simulink model "Lev_project_control_coop_obs"  (R2022b)
settings: Solver=VariableStepAuto  StartTime=0.0  StopTime=Tsim  FixedStep=0.001  RelTol=1e-3
values from neighbouring files (symbols this model uses):
  A = A-B*K0    [project.m]
  Ad = zeros(6,6)    [project.m]
  B = [0; -9.9453]    [project.m]
  C = [708.27 0]    [project.m]
  c = 1/(2*real(minimum_eig))    [project.m]
  D = 0    [project.m]
  G = diag([0 1 0 6 0 0])    [project.m]
  K = (R\B')*P    [project.m]
  x_0 = [0 0]'    [project.m]
  x_0_Leader = [0 2]'    [project.m]
undefined symbols (not defined in the file or in its folder): observer
libraries: matrix_library x6
settings Model: Creator=Matteo  LastModifiedBy=Soff

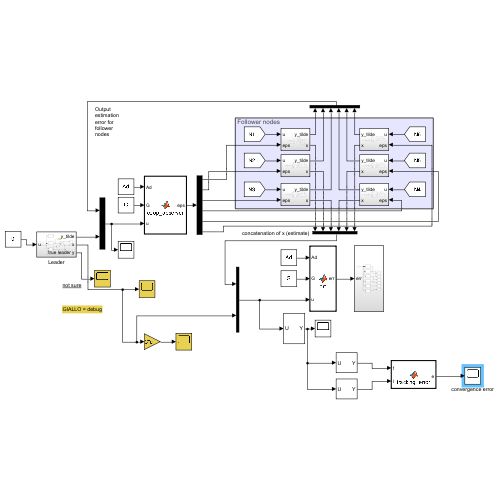
[thumbnail: Simulink's stored preview of the top-level diagram]
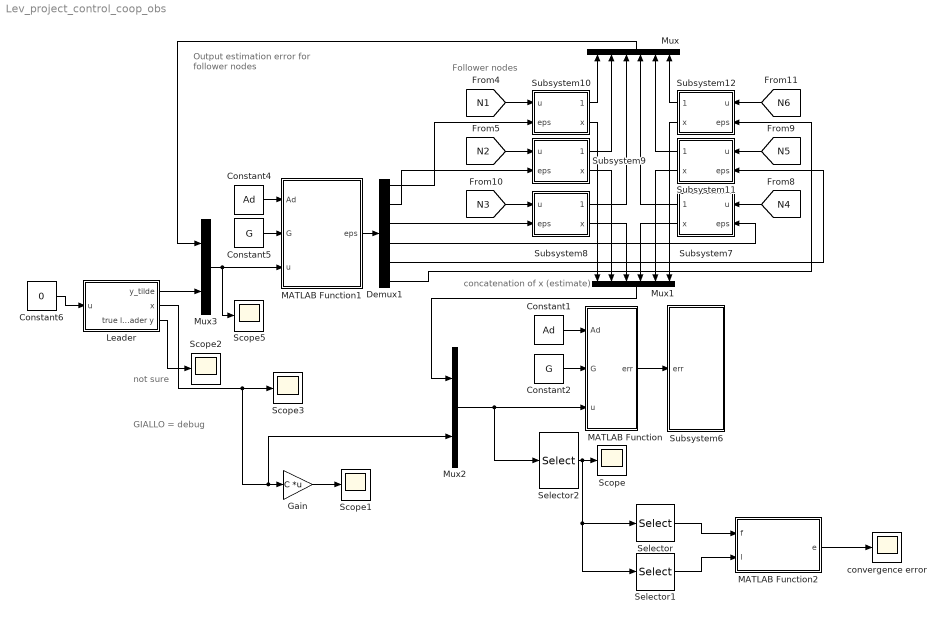
== system Lev_project_control_coop_obs ==
  note: GIALLO = debug
  note: concatenation of x (estimate)
  note: Follower nodes
  note: not sure
  note: Output estimation error for follower nodes
  Constant1 : Constant  Value=Ad
  Constant2 : Constant  Value=G
  Constant4 : Constant  Value=Ad
  Constant5 : Constant  Value=G
  Constant6 : Constant  Value=0
  Demux1 : Demux  Outputs=6
  Gain : Gain  Gain=C  Multiplication=Matrix(K*u)
  Leader : Subsystem
  MATLAB Function : MATLAB Function  TreatAsAtomicUnit=on
  MATLAB Function1 : MATLAB Function  TreatAsAtomicUnit=on
  MATLAB Function2 : MATLAB Function  TreatAsAtomicUnit=on
  Mux : Mux  Inputs=6
  Mux1 : Mux  Inputs=6
  Mux2 : Mux  Inputs=2
  Mux3 : Mux  Inputs=2
  Scope{,1..3,5} (5 alike) : Scope
  Selector : Selector  InputPortWidth=7  IndexOptions=Index vector (dialog)  Indices=[1 2 3 4 5 6]  OutputSizes=1
  Selector1 : Selector  InputPortWidth=7  IndexOptions=Index vector (dialog)  Indices=[7]  OutputSizes=1
  Selector2 : Selector  InputPortWidth=14  IndexOptions=Index vector (dialog)  Indices=[1 3 5 7 9 11 13]  OutputSizes=1
  Subsystem10 : Subsystem
  Subsystem11 : Subsystem
  Subsystem12 : Subsystem
  Subsystem6 : Subsystem
  Subsystem7 : Subsystem
  Subsystem8 : Subsystem
  Subsystem9 : Subsystem
  convergence error : Scope
  wires:
  Constant1/1 -> MATLAB Function/1(Ad)
  Constant2/1 -> MATLAB Function/2(G)
  Constant4/1 -> MATLAB Function1/1(Ad)
  Constant5/1 -> MATLAB Function1/2(G)
  MATLAB Function1/1(eps) -> Demux1/1
  Constant6/1 -> Leader/1(u)
  Mux3/1 -> Scope5/1, MATLAB Function1/3(u)
  Leader/2(x) -> Mux2/2, Gain/1, Scope3/1
  Mux2/1 -> Selector2/1, MATLAB Function/3(u)
  Gain/1 -> Scope1/1
  Leader/3(true leader y) -> Scope2/1
  MATLAB Function/1(err) -> Subsystem6/1(err)
  [N1] -> Subsystem10/1(u)
  [N4] -> Subsystem7/1(u)
  [N2] -> Subsystem9/1(u)
  [N3] -> Subsystem8/1(u)
  [N5] -> Subsystem11/1(u)
  [N6] -> Subsystem12/1(u)
  Subsystem10/1(y_tilde) -> Mux/1
  Subsystem9/1(y_tilde) -> Mux/2
  Subsystem8/1(y_tilde) -> Mux/3
  Subsystem12/1(y_tilde) -> Mux/6
  Subsystem11/1(y_tilde) -> Mux/5
  Subsystem7/1(y_tilde) -> Mux/4
  Demux1/1 -> Subsystem10/2(eps)
  Demux1/3 -> Subsystem8/2(eps)
  Mux/1 -> Mux3/1
  Subsystem10/2(x) -> Mux1/1
  Subsystem9/2(x) -> Mux1/2
  Subsystem8/2(x) -> Mux1/3
  Subsystem7/2(x) -> Mux1/4
  Subsystem11/2(x) -> Mux1/5
  Subsystem12/2(x) -> Mux1/6
  Mux1/1 -> Mux2/1
  Demux1/2 -> Subsystem9/2(eps)
  Demux1/4 -> Subsystem7/2(eps)
  Demux1/5 -> Subsystem11/2(eps)
  Demux1/6 -> Subsystem12/2(eps)
  Leader/1(y_tilde) -> Mux3/2
  Selector2/1 -> Selector/1, Selector1/1, Scope/1
  MATLAB Function2/1(e) -> convergence error/1
  Selector1/1 -> MATLAB Function2/2(l)
  Selector/1 -> MATLAB Function2/1(f)

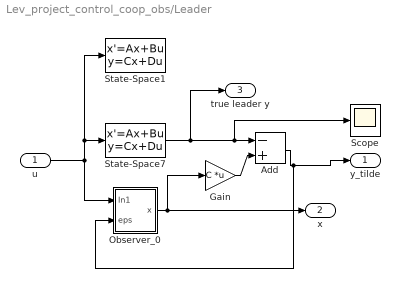
== system Lev_project_control_coop_obs/Leader ==
  u : Inport
  Add : Sum  Inputs=-+
  Gain : Gain  Gain=C  Multiplication=Matrix(K*u)
  Observer_0 : Subsystem
  Scope : Scope
  State-Space1 : StateSpace  A=A  B=B  C=eye(2)  D=zeros(2,1)  InitialCondition=x_0_Leader
  State-Space7 : StateSpace  A=A  B=B  C=C  D=D  InitialCondition=x_0_Leader
  y_tilde : Outport
  x : Outport  Port=2
  true leader y : Outport  Port=3
  wires:
  State-Space7/1 -> Scope/1, Add/1, true leader y/1
  u/1 -> State-Space1/1, State-Space7/1, Observer_0/1(In1)
  Add/1 -> Observer_0/2(eps), y_tilde/1
  Gain/1 -> Add/2
  Observer_0/1(x) -> x/1, Gain/1

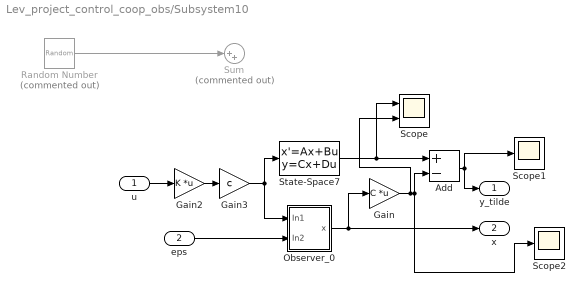
== system Lev_project_control_coop_obs/Subsystem10 ==
  u : Inport
  eps : Inport  Port=2
  Add : Sum  Inputs=+-
  Gain : Gain  Gain=C  Multiplication=Matrix(K*u)
  Gain2 : Gain  Gain=K  Multiplication=Matrix(K*u)
  Gain3 : Gain  Gain=c
  Observer_0 : Subsystem
  Random Number : RandomNumber  Commented=on  SampleTime=0.1
  Scope : Scope  NumInputPorts=2
  Scope1 : Scope
  Scope2 : Scope
  State-Space7 : StateSpace  A=A  B=B  C=C  D=D  InitialCondition=x_0
  Sum : Sum  Commented=on  Inputs=|++
  y_tilde : Outport
  x : Outport  Port=2
  wires:
  Gain/1 -> Scope/2, Add/2, Scope2/1
  Add/1 -> y_tilde/1, Scope1/1
  eps/1 -> Observer_0/2(In2)
  Observer_0/1(x) -> x/1, Gain/1
  u/1 -> Gain2/1
  Gain2/1 -> Gain3/1
  Gain3/1 -> Observer_0/1(In1), State-Space7/1
  Random Number/1 -> Sum/1
  State-Space7/1 -> Scope/1, Add/1

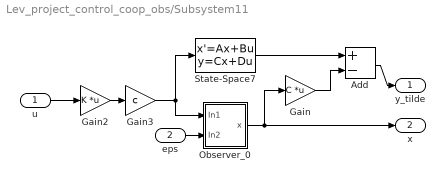
== system Lev_project_control_coop_obs/Subsystem11 ==
  u : Inport
  eps : Inport  Port=2
  Add : Sum  Inputs=+-
  Gain : Gain  Gain=C  Multiplication=Matrix(K*u)
  Gain2 : Gain  Gain=K  Multiplication=Matrix(K*u)
  Gain3 : Gain  Gain=c
  Observer_0 : Subsystem
  State-Space7 : StateSpace  A=A  B=B  C=C  D=D  InitialCondition=x_0
  y_tilde : Outport
  x : Outport  Port=2
  wires:
  u/1 -> Gain2/1
  Add/1 -> y_tilde/1
  Gain/1 -> Add/2
  State-Space7/1 -> Add/1
  Observer_0/1(x) -> x/1, Gain/1
  eps/1 -> Observer_0/2(In2)
  Gain2/1 -> Gain3/1
  Gain3/1 -> Observer_0/1(In1), State-Space7/1

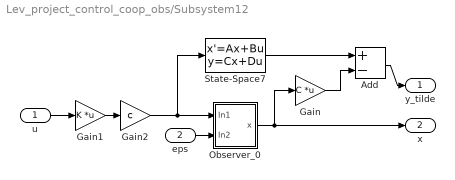
== system Lev_project_control_coop_obs/Subsystem12 ==
  u : Inport
  eps : Inport  Port=2
  Add : Sum  Inputs=+-
  Gain : Gain  Gain=C  Multiplication=Matrix(K*u)
  Gain1 : Gain  Gain=K  Multiplication=Matrix(K*u)
  Gain2 : Gain  Gain=c
  Observer_0 : Subsystem
  State-Space7 : StateSpace  A=A  B=B  C=C  D=D  InitialCondition=x_0
  y_tilde : Outport
  x : Outport  Port=2
  wires:
  Add/1 -> y_tilde/1
  Gain/1 -> Add/2
  State-Space7/1 -> Add/1
  Observer_0/1(x) -> x/1, Gain/1
  eps/1 -> Observer_0/2(In2)
  Gain1/1 -> Gain2/1
  Gain2/1 -> Observer_0/1(In1), State-Space7/1
  u/1 -> Gain1/1

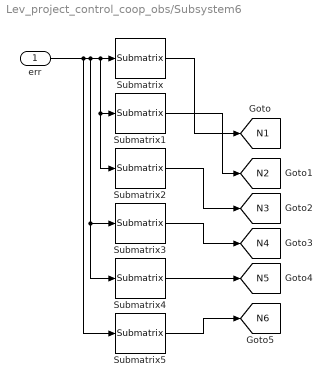
== system Lev_project_control_coop_obs/Subsystem6 ==
  err : Inport
  Submatrix : matrix_library/Submatrix  RowSpan=All rows  RowStartMode=First  RowStartIndex=1  RowEndMode=Last  RowEndIndex=1  ColSpan=One column  ColStartMode=Index  ColStartIndex=1  ColEndMode=Last  ColEndIndex=1
  Submatrix1 : matrix_library/Submatrix  RowSpan=All rows  RowStartMode=First  RowStartIndex=1  RowEndMode=Last  RowEndIndex=1  ColSpan=One column  ColStartMode=Index  ColStartIndex=2  ColEndMode=Last  ColEndIndex=1
  Submatrix2 : matrix_library/Submatrix  RowSpan=All rows  RowStartMode=First  RowStartIndex=1  RowEndMode=Last  RowEndIndex=1  ColSpan=One column  ColStartMode=Index  ColStartIndex=3  ColEndMode=Last  ColEndIndex=1
  Submatrix3 : matrix_library/Submatrix  RowSpan=All rows  RowStartMode=First  RowStartIndex=1  RowEndMode=Last  RowEndIndex=1  ColSpan=One column  ColStartMode=Index  ColStartIndex=4  ColEndMode=Last  ColEndIndex=1
  Submatrix4 : matrix_library/Submatrix  RowSpan=All rows  RowStartMode=First  RowStartIndex=1  RowEndMode=Last  RowEndIndex=1  ColSpan=One column  ColStartMode=Index  ColStartIndex=5  ColEndMode=Last  ColEndIndex=1
  Submatrix5 : matrix_library/Submatrix  RowSpan=All rows  RowStartMode=First  RowStartIndex=1  RowEndMode=Last  RowEndIndex=1  ColSpan=One column  ColStartMode=Index  ColStartIndex=6  ColEndMode=Last  ColEndIndex=1
  tag scope: N1=global, N2=global, N3=global, N4=global, N5=global, N6=global
  wires:
  Submatrix4/1 -> [N5]
  Submatrix/1 -> [N1]
  Submatrix3/1 -> [N4]
  err/1 -> Submatrix5/1, Submatrix3/1, Submatrix4/1, Submatrix1/1, Submatrix2/1, Submatrix/1
  Submatrix5/1 -> [N6]
  Submatrix2/1 -> [N3]
  Submatrix1/1 -> [N2]

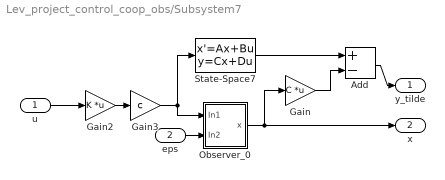
== system Lev_project_control_coop_obs/Subsystem7 ==
  u : Inport
  eps : Inport  Port=2
  Add : Sum  Inputs=+-
  Gain : Gain  Gain=C  Multiplication=Matrix(K*u)
  Gain2 : Gain  Gain=K  Multiplication=Matrix(K*u)
  Gain3 : Gain  Gain=c
  Observer_0 : Subsystem
  State-Space7 : StateSpace  A=A  B=B  C=C  D=D  InitialCondition=x_0
  y_tilde : Outport
  x : Outport  Port=2
  wires:
  Add/1 -> y_tilde/1
  Gain/1 -> Add/2
  State-Space7/1 -> Add/1
  Observer_0/1(x) -> x/1, Gain/1
  eps/1 -> Observer_0/2(In2)
  Gain2/1 -> Gain3/1
  u/1 -> Gain2/1
  Gain3/1 -> Observer_0/1(In1), State-Space7/1

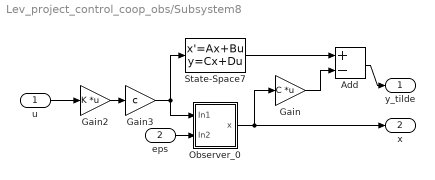
== system Lev_project_control_coop_obs/Subsystem8 ==
  u : Inport
  eps : Inport  Port=2
  Add : Sum  Inputs=+-
  Gain : Gain  Gain=C  Multiplication=Matrix(K*u)
  Gain2 : Gain  Gain=K  Multiplication=Matrix(K*u)
  Gain3 : Gain  Gain=c
  Observer_0 : Subsystem
  State-Space7 : StateSpace  A=A  B=B  C=C  D=D  InitialCondition=x_0
  y_tilde : Outport
  x : Outport  Port=2
  wires:
  Add/1 -> y_tilde/1
  Gain/1 -> Add/2
  State-Space7/1 -> Add/1
  Observer_0/1(x) -> x/1, Gain/1
  eps/1 -> Observer_0/2(In2)
  Gain2/1 -> Gain3/1
  u/1 -> Gain2/1
  Gain3/1 -> Observer_0/1(In1), State-Space7/1

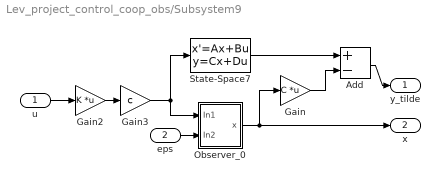
== system Lev_project_control_coop_obs/Subsystem9 ==
  u : Inport
  eps : Inport  Port=2
  Add : Sum  Inputs=+-
  Gain : Gain  Gain=C  Multiplication=Matrix(K*u)
  Gain2 : Gain  Gain=K  Multiplication=Matrix(K*u)
  Gain3 : Gain  Gain=c
  Observer_0 : Subsystem
  State-Space7 : StateSpace  A=A  B=B  C=C  D=D  InitialCondition=x_0
  y_tilde : Outport
  x : Outport  Port=2
  wires:
  Add/1 -> y_tilde/1
  Gain/1 -> Add/2
  State-Space7/1 -> Add/1
  Observer_0/1(x) -> x/1, Gain/1
  eps/1 -> Observer_0/2(In2)
  Gain2/1 -> Gain3/1
  u/1 -> Gain2/1
  Gain3/1 -> Observer_0/1(In1), State-Space7/1

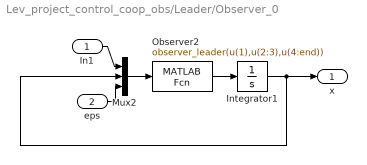
== system Lev_project_control_coop_obs/Leader/Observer_0 ==
  In1 : Inport
  eps : Inport  Port=2
  Integrator1 : Integrator  InitialCondition=[0;0]
  Mux2 : Mux  Inputs=3
  Observer2 : MATLABFcn  MATLABFcn=observer_leader(u(1),u(2:3),u(4:end))
  x : Outport
  wires:
  Integrator1/1 -> x/1, Mux2/2
  Mux2/1 -> Observer2/1
  Observer2/1 -> Integrator1/1
  eps/1 -> Mux2/3
  In1/1 -> Mux2/1

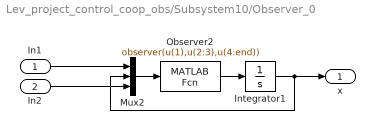
== system Lev_project_control_coop_obs/Subsystem10/Observer_0 ==
  In1 : Inport
  In2 : Inport  Port=2
  Integrator1 : Integrator  InitialCondition=[0;0]
  Mux2 : Mux  Inputs=3
  Observer2 : MATLABFcn  MATLABFcn=observer(u(1),u(2:3),u(4:end))
  x : Outport
  wires:
  Integrator1/1 -> x/1, Mux2/2
  Mux2/1 -> Observer2/1
  Observer2/1 -> Integrator1/1
  In2/1 -> Mux2/3
  In1/1 -> Mux2/1

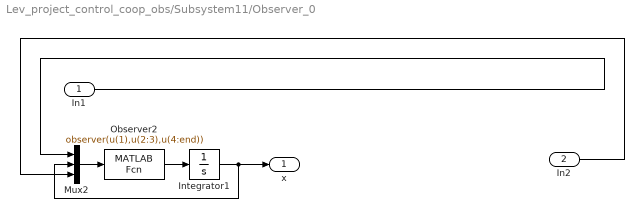
== system Lev_project_control_coop_obs/Subsystem11/Observer_0 ==
  In1 : Inport
  In2 : Inport  Port=2
  Integrator1 : Integrator  InitialCondition=[0;0]
  Mux2 : Mux  Inputs=3
  Observer2 : MATLABFcn  MATLABFcn=observer(u(1),u(2:3),u(4:end))
  x : Outport
  wires:
  Integrator1/1 -> x/1, Mux2/2
  Mux2/1 -> Observer2/1
  Observer2/1 -> Integrator1/1
  In2/1 -> Mux2/3
  In1/1 -> Mux2/1

== system Lev_project_control_coop_obs/Subsystem12/Observer_0 ==
  In1 : Inport
  In2 : Inport  Port=2
  Integrator1 : Integrator  InitialCondition=[0;0]
  Mux2 : Mux  Inputs=3
  Observer2 : MATLABFcn  MATLABFcn=observer(u(1),u(2:3),u(4:end))
  x : Outport
  wires:
  Integrator1/1 -> x/1, Mux2/2
  Mux2/1 -> Observer2/1
  Observer2/1 -> Integrator1/1
  In2/1 -> Mux2/3
  In1/1 -> Mux2/1

== system Lev_project_control_coop_obs/Subsystem7/Observer_0 ==
  In1 : Inport
  In2 : Inport  Port=2
  Integrator1 : Integrator  InitialCondition=[0;0]
  Mux2 : Mux  Inputs=3
  Observer2 : MATLABFcn  MATLABFcn=observer(u(1),u(2:3),u(4:end))
  x : Outport
  wires:
  Integrator1/1 -> x/1, Mux2/2
  Mux2/1 -> Observer2/1
  Observer2/1 -> Integrator1/1
  In1/1 -> Mux2/1
  In2/1 -> Mux2/3

== system Lev_project_control_coop_obs/Subsystem8/Observer_0 ==
  In1 : Inport
  In2 : Inport  Port=2
  Integrator1 : Integrator  InitialCondition=[0;0]  UpperSaturationLimit=1e6  LowerSaturationLimit=-1e6
  Mux2 : Mux  Inputs=3
  Observer2 : MATLABFcn  MATLABFcn=observer(u(1),u(2:3),u(4))
  x : Outport
  wires:
  Integrator1/1 -> x/1, Mux2/2
  Mux2/1 -> Observer2/1
  Observer2/1 -> Integrator1/1
  In2/1 -> Mux2/3
  In1/1 -> Mux2/1

== system Lev_project_control_coop_obs/Subsystem9/Observer_0 ==
  In1 : Inport
  In2 : Inport  Port=2
  Integrator1 : Integrator  InitialCondition=[0;0]
  Mux2 : Mux  Inputs=3
  Observer2 : MATLABFcn  MATLABFcn=observer(u(1),u(2:3),u(4:end))
  x : Outport
  wires:
  Integrator1/1 -> x/1, Mux2/2
  Mux2/1 -> Observer2/1
  Observer2/1 -> Integrator1/1
  In2/1 -> Mux2/3
  In1/1 -> Mux2/1

== matlab function Lev_project_control_coop_obs/MATLAB Function1 ==
  data: Ad input; G input; u input; eps output
function eps = coop_observer(Ad,G,u)

% output dimension (single node)
n = 1;

% number of follower nodes
m = 6;

x=zeros(n,m+1);
tmp = u';

for j = 1:m+1
    for i = 1:n
        x(i,j) = tmp(1);
        tmp = circshift(tmp,[0 -1]);
    end
end
% Column i = output error of node i (m+1 for leader)

eps = zeros(n,m);
for i = 1:m
    for j = 1:m
        if i ~= j
            eps(:,i) = eps(:,i) + Ad(i,j)*(x(:,j)-x(:,i));
        end
    end
    
    eps(:,i) = eps(:,i) + G(i,j)*(x(:,m+1)-x(:,i));
end

== matlab function Lev_project_control_coop_obs/MATLAB Function ==
  data: Ad input; G input; u input; err output
function err = err(Ad,G,u)

% state dimension (single node)
n = 2;

% number of follower nodes
m = 6;

x=zeros(n,m+1);

tmp = u';

for j = 1:m+1
    for i = 1:n
        x(i,j) = tmp(1);
        tmp = circshift(tmp,[0 -1]);
    end
%     x(:,j)
end

err = zeros(n, m);

for i = 1:m
    for j = 1:m
        err(:, i) = err(:, i) + Ad(i, j) * (x(:, j) - x(:, i));
    end

    err(:, i) = err(:, i) + G(i, i) * (x(:, m + 1) - x(:, i));
end

== matlab function Lev_project_control_coop_obs/MATLAB Function2 ==
  data: f input; e output; l input
function e = tracking_error(f, l)

e = zeros(6, size(l,2));
l_mat = l*ones(6, size(l, 2));
e(1:6,:) = l_mat - f(1:6,:);

end
